simulink model "Test_IGBT_Diode"  (R2024a)
settings: Solver=VariableStepAuto  StartTime=0.0  StopTime=20e-6  RelTol=1e-3
libraries: spsDiodeLib x2, spsIGBTLib x2, spsGroundLib x1, spsControlledCurrentSourceLib x1, spsCurrentMeasurementLib x1, spsVoltageMeasurementLib x1, spsDCVoltageSourceLib x1, sps_lib x1
settings Model: Creator=nothi  LastModifiedBy=nothi

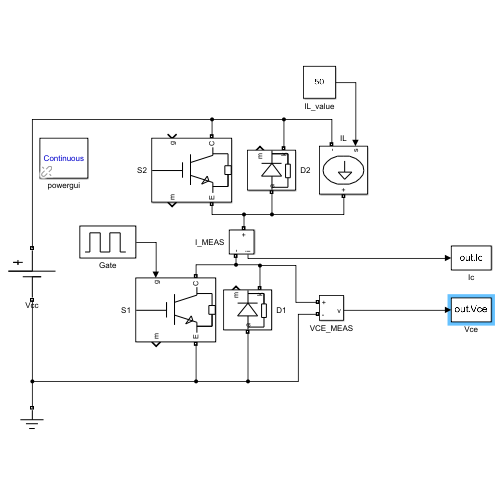
[thumbnail: Simulink's stored preview of the top-level diagram]
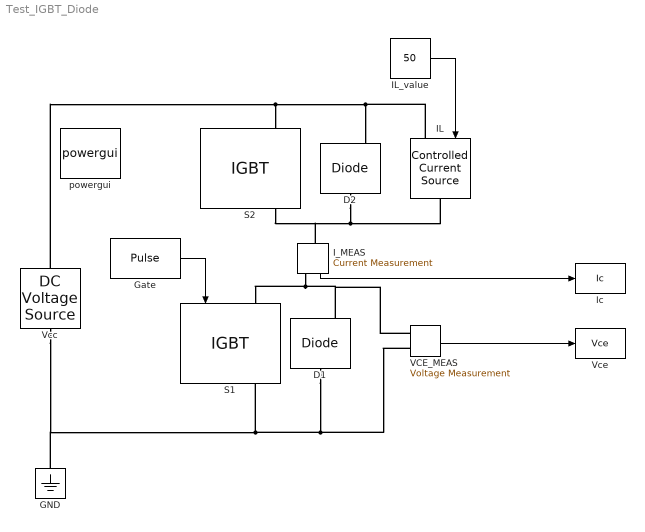
== system Test_IGBT_Diode ==
  D1 : spsDiodeLib/Diode  Ron=0.001  Lon=0  Vf=0.8  IC=0  UseSnubber=0  Rs=500  Cs=250e-9  Measurements=on
  D2 : spsDiodeLib/Diode  Ron=0.001  Lon=0  Vf=0.8  IC=0  UseSnubber=0  Rs=500  Cs=250e-9  Measurements=on
  GND : spsGroundLib/Ground  LConnTagsString=a
  Gate : DiscretePulseGenerator  PulseType=Time based  Amplitude=15  Period=5e-6  PulseWidth=50
  IL : spsControlledCurrentSourceLib/Controlled Current Source  Initialize=on  Source_Type=AC  Amplitude=50  Phase=0  Frequency=0  Measurements=None
  IL_value : Constant  Value=50
  I_MEAS : spsCurrentMeasurementLib/Current Measurement  PhasorSimulation=off  OutputType=Complex  PSBequivalent=0
  Ic : ToWorkspace  VariableName=Ic  SaveFormat=Structure With Time  SampleTime=-1
  S1 : spsIGBTLib/IGBT  Ron=0.001  Lon=0  Vf=1  Tf=1e-6  Tt=2e-6  IC=0  Rs=1e5  Cs=inf  Measurements=on
  S2 : spsIGBTLib/IGBT  Ron=0.001  Lon=0  Vf=1  Tf=1e-6  Tt=2e-6  IC=0  Rs=1e5  Cs=inf  Measurements=on
  VCE_MEAS : spsVoltageMeasurementLib/Voltage Measurement  PhasorSimulation=off  OutputType=Complex  PSBequivalent=0
  Vcc : spsDCVoltageSourceLib/DC Voltage Source  Amplitude=500  Measurements=None
  Vce : ToWorkspace  VariableName=Vce  SaveFormat=Structure With Time  SampleTime=-1
  powergui : sps_lib/powergui  Priority=1  SimulationMode=Continuous  SampleTime=50e-6  frequency=60  Iterations=50  frequencyindice=0  Pbase=100e6  ErrMax=1e-4  UnitsV=kV  UnitsW=MW  buscounter=0  FunctionMessages=off  echomessages=off  EnableUseOfTLC=off  CurrentSourceSwitches=off  DisableSnubberDevices=off  DisableRonSwitches=off  DisableVfSwitches=off  DisplayEquations=off  AutomaticDiscreteSolvers=off  SolverType=Tustin/Backward Euler (TBE)  Interpol=off  ExternalGateDelay=off  methode=off  Ts=100  x0status=blocks  SPID=on  SwTol=0  HookPort=off  NonlinearTolerance=1e-4  nMaxIteration=100  ContinueOnMaxIteration=off  RestoreLinks=warning  ResistiveCurrentMeasurement=off  Frange=[0:2:500]  Ylog=off  Xlog=on  ShowGrid=off  save=off  variable=ZData  structure=0  ZoomFFT=off  StartTime=0.0  cycles=1  DisplayStyle=1  fundamental=60  FreqAxis=off  MaxFrequency=1000  frequencyindicesteady=1  RmsSteady=1  display=off
  wires:
  IL_value/1 -> IL/1
  Gate/1 -> S1/1
  VCE_MEAS/1 -> Vce/1
  I_MEAS/1 -> Ic/1
  connections:
  Vcc/RConn1 -- IL/LConn1 -- D2/RConn1 -- S2/LConn1
  D2/LConn1 -- IL/RConn1 -- S2/RConn1 -- I_MEAS/LConn1
  D1/LConn1 -- VCE_MEAS/LConn2 -- S1/RConn1 -- Vcc/LConn1 -- GND/LConn1
  I_MEAS/RConn1 -- VCE_MEAS/LConn1 -- D1/RConn1 -- S1/LConn1
